simulink model "observer"  (R2019a)
settings: Solver=ode45  StartTime=0.0  StopTime=10.0  RelTol=1e-3
values from neighbouring files (symbols this model uses):
  A = [0, 1, 0, 0 ... (first row only)    [lab.m]
  B = [0 ... (first row only)    [lab.m]
  C = [1, 0, 0, 0 ... (first row only)    [lab.m]
  F = -acker(A, B, eign_F)    [lab.m]
  K = K2    [lab.m]
undefined symbols (not defined in the file or in its folder): A1
settings Model: Creator=ZIXUANXU  LastModifiedBy=ZIXUANXU
settings DataIOCC: ReturnWorkspaceOutputs=off  Refine=4

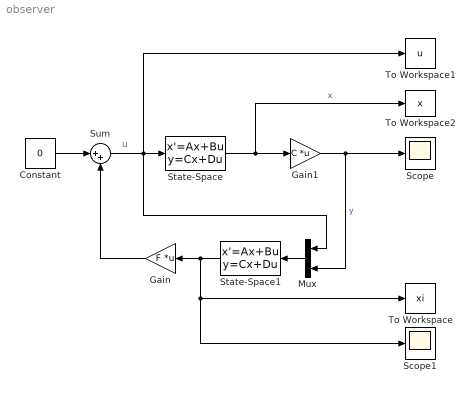
== system observer ==
  note: u
  Constant : Constant  Value=0
  Gain : Gain  Gain=F  Multiplication=Matrix(K*u)
  Gain1 : Gain  Gain=C  Multiplication=Matrix(K*u)
  Mux : Mux  Inputs=2
  Scope : Scope
  Scope1 : Scope
  State-Space : StateSpace  A=A  B=B  C=eye(4)  D=zeros(4,1)  InitialCondition=[0.1 0 0.1 0]
  State-Space1 : StateSpace  A=A1  B=[B K]  C=eye(4)  D=zeros(4, 3)  InitialCondition=[0 0 0 0]
  Sum : Sum  Inputs=|++
  To Workspace : ToWorkspace  VariableName=xi  SampleTime=-1
      settings: Save2DSignal=2-D array (concatenate along first dimension)
  To Workspace1 : ToWorkspace  VariableName=u  SampleTime=-1
      settings: Save2DSignal=2-D array (concatenate along first dimension)
  To Workspace2 : ToWorkspace  VariableName=x  SampleTime=-1
      settings: Save2DSignal=2-D array (concatenate along first dimension)
  wires:
  Constant/1 -> Sum/1
  Sum/1 -> State-Space/1, To Workspace1/1, Mux/1
  State-Space/1 -> Gain1/1, To Workspace2/1  "x"
  Mux/1 -> State-Space1/1
  State-Space1/1 -> Scope1/1, To Workspace/1, Gain/1
  Gain/1 -> Sum/2
  Gain1/1 -> Mux/2, Scope/1  "y"
